simulink model "Task4_sim"  (R2014a)
settings: Solver=ode45  StartTime=0.0  StopTime=0.3  RelTol=1e-3
settings Model: Creator=bunka  LastModifiedBy=bunka

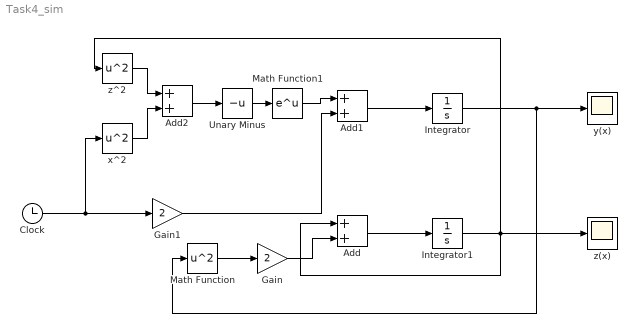
== system Task4_sim ==
  Add : Sum
  Add1 : Sum
  Add2 : Sum
  Clock : Clock
  Gain : Gain  Gain=2
  Gain1 : Gain  Gain=2
  Integrator : Integrator  InitialCondition=0.5
  Integrator1 : Integrator  InitialCondition=1
  Math Function : Math  Operator=square  SaturateOnIntegerOverflow=on
  Math Function1 : Math  SaturateOnIntegerOverflow=on
  Unary Minus : UnaryMinus
  x^2 : Math  Operator=square  SaturateOnIntegerOverflow=on
  y(x) : Scope
  z(x) : Scope
  z^2 : Math  Operator=square  SaturateOnIntegerOverflow=on
  wires:
  Integrator/1 -> Math Function/1, y(x)/1
  Integrator1/1 -> z(x)/1, z^2/1, Add/1
  Add/1 -> Integrator1/1
  Gain/1 -> Add/2
  Math Function/1 -> Gain/1
  Add1/1 -> Integrator/1
  Unary Minus/1 -> Math Function1/1
  Add2/1 -> Unary Minus/1
  x^2/1 -> Add2/2
  z^2/1 -> Add2/1
  Clock/1 -> Gain1/1, x^2/1
  Math Function1/1 -> Add1/1
  Gain1/1 -> Add1/2
